simulink model "TestSeqAndDMS_Master"  (R2015b)
settings: Solver=FixedStepDiscrete  SolverMode=SingleTasking  StartTime=0.0  StopTime=inf  RelTol=1e-3
PreLoadFcn:
  | addpath RealTime_Pacer
PostLoadFcn:
  | StimuliImport
libraries: Word2Bytes_lib x41, simulink x3, instrumentlib x3, epoch_time_lib x2, realtime_pacer_lib x1
settings Model: Creator=ch24070  LastModifiedBy=ED12083
settings DataIOCC: LimitDataPoints=off  SaveFormat=StructureWithTime
settings DebuggingCC: SFUnexpectedBacktrackingDiag=error  SFNoUnconditionalDefaultTransitionDiag=error
settings HardwareCC: ProdWordSize=32  ProdHWDeviceType=Specified
settings ModelReferenceCC: PropagateSignalLabelsOutOfModel=on
settings GRTTargetCC: TargetLangStandard=C99 (ISO)
settings ConfigComp: CovMetricSettings=dwe  CovHtmlReporting=off  CovSaveCumulativeToWorkspaceVar=off  CovSaveSingleToWorkspaceVar=off  CovModelRefEnable=Off  CovExternalEMLEnable=on

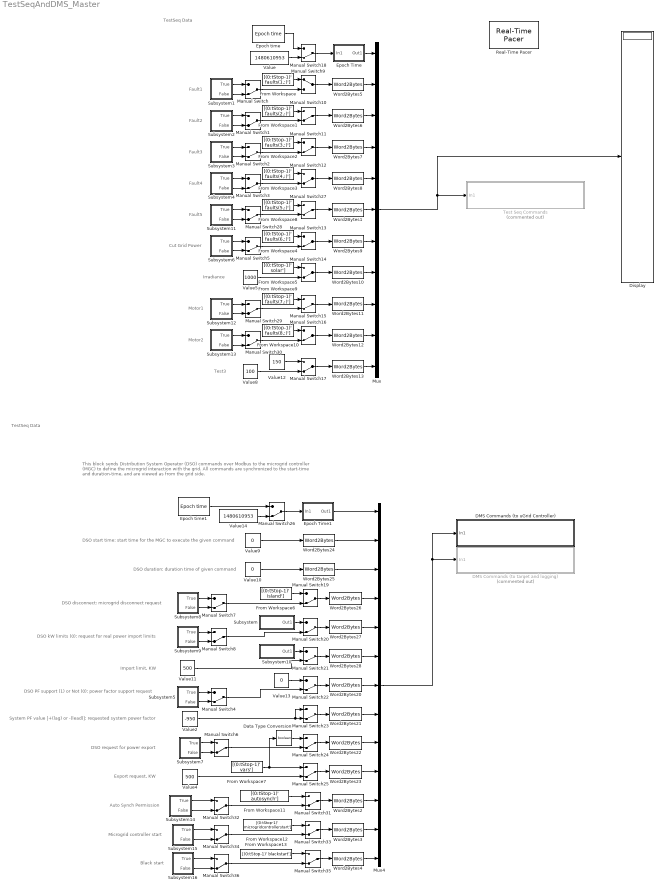
== system TestSeqAndDMS_Master ==
  note: Fault1
  note: This block sends Distribution System Operator (DSO) commands over Modbus to the microgrid controller (MGC) to define the microgrid
      | interaction with the grid. All commands are synchronized to the start-time and duration-time, and are viewed as from the grid side.
  note: TestSeq Data
  note: Fault2
  note: Fault3
  note: Fault4
  note: Cut Grid Power
  note: Irradiance
  note: Motor1
  note: Motor2
  note: Test3
  note: DSO disconnect: microgrid disconnect request
  note: DSO kW limits (0): request for real power import limits
  note: Import limit, KW
  note: DSO PF support (1) or Not (0): power factor support request
  note: System PF value [+(lag) or -(lead)]: requested system power factor
  note: DSO request for power export
  note: Export request, KW
  note: DSO start time: start time for the MGC to execute the given command
  note: DSO duration: duration time of given command
  note: Fault5
  note: Auto Synch Permission
  note: Microgrid controller start
  note: Black start
  note: TestSeq Data
  DMS Commands (to target and logging) : Subsystem  Commented=on  mask{destIP='192.168.10.54', unitID=54, modAddr=2000}
      mask prompts: destIP "Destination IP"; modAddr "Modbus Starting Address"
      mask Display:
      | text(5, 40, 'Modbus Master Write Holding Registers');
      | text(5, 20, ['Dest IP: ' destIP]);
  DMS Commands (to uGrid Controller) : Subsystem  mask{destIP='10.10.45.19', unitID=1, modAddr=2000}
      mask prompts: destIP "Destination IP"; modAddr "Modbus Starting Address"
      mask Display:
      | text(5, 40, 'Modbus Master Write Holding Registers');
      | text(5, 20, ['Dest IP: ' destIP]);
  Data Type Conversion : DataTypeConversion  OutDataTypeStr=boolean
  Display : Display
  Epoch Time : Subsystem
  Epoch Time1 : Subsystem
  Epoch time : epoch_time_lib/Epoch time  syncRate=10  clkRate=1
  Epoch time1 : epoch_time_lib/Epoch time  syncRate=10  clkRate=1
  From Workspace : FromWorkspace  VariableName=[(0:tStop-1)' faults(1,:)']  SampleTime=1  OutputAfterFinalValue=Holding final value
  From Workspace1 : FromWorkspace  VariableName=[(0:tStop-1)' faults(2,:)']  SampleTime=1  OutputAfterFinalValue=Holding final value
  From Workspace10 : FromWorkspace  VariableName=[(0:tStop-1)' faults(8,:)']  SampleTime=1  OutputAfterFinalValue=Holding final value
  From Workspace11 : FromWorkspace  VariableName=[(0:tStop-1)' autosynch']  SampleTime=1  OutputAfterFinalValue=Holding final value
  From Workspace12 : FromWorkspace  VariableName=[(0:tStop-1)' microgridcontrollerstart']  SampleTime=1  OutputAfterFinalValue=Holding final value
  From Workspace13 : FromWorkspace  VariableName=[(0:tStop-1)' blackstart']  SampleTime=1  OutputAfterFinalValue=Holding final value
  From Workspace2 : FromWorkspace  VariableName=[(0:tStop-1)' faults(3,:)']  SampleTime=1  OutputAfterFinalValue=Holding final value
  From Workspace3 : FromWorkspace  VariableName=[(0:tStop-1)' faults(4,:)']  SampleTime=1  OutputAfterFinalValue=Holding final value
  From Workspace4 : FromWorkspace  VariableName=[(0:tStop-1)' faults(6,:)']  SampleTime=1  OutputAfterFinalValue=Holding final value
  From Workspace5 : FromWorkspace  VariableName=[(0:tStop-1)' solar']  SampleTime=1  OutputAfterFinalValue=Holding final value
  From Workspace6 : FromWorkspace  VariableName=[(0:tStop-1)' island']  SampleTime=1  OutputAfterFinalValue=Holding final value
  From Workspace7 : FromWorkspace  VariableName=[(0:tStop-1)' vars']  SampleTime=1  OutputAfterFinalValue=Holding final value
  From Workspace8 : FromWorkspace  VariableName=[(0:tStop-1)' faults(5,:)']  SampleTime=1  OutputAfterFinalValue=Holding final value
  From Workspace9 : FromWorkspace  VariableName=[(0:tStop-1)' faults(7,:)']  SampleTime=1  OutputAfterFinalValue=Holding final value
  Manual Switch{,1..8,10..36} (36 alike) : ManualSwitch  CurrentSetting=0
  Manual Switch9 : ManualSwitch
  Mux : Mux  Inputs=11
  Mux4 : Mux  Inputs=13
  Real-Time Pacer : realtime_pacer_lib/Real-Time Pacer  simTimePerRealTime=1
  Subsystem : Subsystem
  Subsystem1 : Subsystem
  Subsystem10 : Subsystem
  Subsystem11 : Subsystem
  Subsystem12 : Subsystem
  Subsystem13 : Subsystem
  Subsystem14 : Subsystem
  Subsystem15 : Subsystem
  Subsystem16 : Subsystem
  Subsystem2 : Subsystem
  Subsystem3 : Subsystem
  Subsystem4 : Subsystem
  Subsystem5 : Subsystem
  Subsystem6 : Subsystem
  Subsystem7 : Subsystem
  Subsystem8 : Subsystem
  Subsystem9 : Subsystem
  Test Seq Commands : Subsystem  Commented=on  mask{destIP='192.168.10.56', unitID=56, modAddr=2000}
      mask prompts: destIP "Destination IP"; modAddr "Modbus Starting Address"
      mask Display:
      | text(5, 40, 'Modbus Master Write Holding Registers');
      | text(5, 20, ['Dest IP: ' destIP]);
  Value : Constant  Value=1480610953  OutDataTypeStr=uint32
  Value10 : Constant  Value=0  OutDataTypeStr=uint16
  Value11 : Constant  Value=500  OutDataTypeStr=uint16
  Value12 : Constant  Value=150  OutDataTypeStr=uint16
  Value13 : Constant  Value=0  OutDataTypeStr=uint16
  Value14 : Constant  Value=1480610953  OutDataTypeStr=uint32
  Value2 : Constant  Value=-950  OutDataTypeStr=int16
  Value4 : Constant  Value=500  OutDataTypeStr=uint16
  Value5 : Constant  Value=1000  OutDataTypeStr=uint16
  Value8 : Constant  Value=100  OutDataTypeStr=uint16
  Value9 : Constant  Value=0  OutDataTypeStr=uint16
  Word2Bytes{1..13,20..28} (22 alike) : Word2Bytes_lib/Word2Bytes
  wires:
  Epoch Time/1(Out1) -> Mux/1
  Subsystem1/2(False) -> Manual Switch/2
  Word2Bytes5/1 -> Mux/2
  Word2Bytes6/1 -> Mux/3
  Word2Bytes7/1 -> Mux/4
  Word2Bytes8/1 -> Mux/5
  Subsystem1/1(True) -> Manual Switch/1
  Subsystem2/2(False) -> Manual Switch1/2
  Subsystem2/1(True) -> Manual Switch1/1
  Subsystem3/2(False) -> Manual Switch2/2
  Subsystem3/1(True) -> Manual Switch2/1
  Subsystem4/1(True) -> Manual Switch3/1
  Subsystem6/2(False) -> Manual Switch5/2
  Subsystem6/1(True) -> Manual Switch5/1
  Subsystem4/2(False) -> Manual Switch3/2
  Epoch Time1/1(Out1) -> Mux4/1
  Value9/1 -> Word2Bytes24/1
  Word2Bytes24/1 -> Mux4/2
  Value10/1 -> Word2Bytes25/1
  Word2Bytes25/1 -> Mux4/3
  Word2Bytes26/1 -> Mux4/4
  Word2Bytes27/1 -> Mux4/5
  Word2Bytes28/1 -> Mux4/6
  Word2Bytes20/1 -> Mux4/7
  Word2Bytes21/1 -> Mux4/8
  Word2Bytes22/1 -> Mux4/9
  Word2Bytes23/1 -> Mux4/10
  Subsystem8/2(False) -> Manual Switch7/2
  Subsystem8/1(True) -> Manual Switch7/1
  Subsystem9/1(True) -> Manual Switch8/1
  Subsystem9/2(False) -> Manual Switch8/2
  Subsystem5/2(False) -> Manual Switch4/2
  Subsystem5/1(True) -> Manual Switch4/1
  Subsystem7/2(False) -> Manual Switch6/2
  Subsystem7/1(True) -> Manual Switch6/1
  Manual Switch9/1 -> Word2Bytes5/1
  Manual Switch/1 -> Manual Switch9/2
  Manual Switch10/1 -> Word2Bytes6/1
  Manual Switch11/1 -> Word2Bytes7/1
  Manual Switch12/1 -> Word2Bytes8/1
  Manual Switch13/1 -> Word2Bytes9/1
  Manual Switch14/1 -> Word2Bytes10/1
  Manual Switch15/1 -> Word2Bytes11/1
  Manual Switch16/1 -> Word2Bytes12/1
  Manual Switch17/1 -> Word2Bytes13/1
  Manual Switch1/1 -> Manual Switch10/2
  Manual Switch2/1 -> Manual Switch11/2
  Manual Switch3/1 -> Manual Switch12/2
  Manual Switch5/1 -> Manual Switch13/2
  Value5/1 -> Manual Switch14/2
  Manual Switch29/1 -> Manual Switch15/2
  Value8/1 -> Manual Switch17/2
  From Workspace/1 -> Manual Switch9/1
  From Workspace1/1 -> Manual Switch10/1
  From Workspace2/1 -> Manual Switch11/1
  From Workspace3/1 -> Manual Switch12/1
  From Workspace4/1 -> Manual Switch13/1
  From Workspace5/1 -> Manual Switch14/1
  Value12/1 -> Manual Switch17/1
  Manual Switch18/1 -> Epoch Time/1(In1)
  Value/1 -> Manual Switch18/2
  Epoch time/1 -> Manual Switch18/1
  Manual Switch19/1 -> Word2Bytes26/1
  From Workspace6/1 -> Manual Switch19/1
  Manual Switch7/1 -> Manual Switch19/2
  Manual Switch20/1 -> Word2Bytes27/1
  Manual Switch8/1 -> Manual Switch20/2
  Subsystem/1(Out1) -> Manual Switch20/1
  Subsystem10/1(Out1) -> Manual Switch21/1
  Manual Switch21/1 -> Word2Bytes28/1
  Value11/1 -> Manual Switch21/2
  Manual Switch22/1 -> Word2Bytes20/1
  Manual Switch4/1 -> Manual Switch22/2
  Value13/1 -> Manual Switch22/1
  Manual Switch23/1 -> Word2Bytes21/1
  Value2/1 -> Manual Switch23/1, Manual Switch23/2
  Manual Switch24/1 -> Word2Bytes22/1
  Manual Switch25/1 -> Word2Bytes23/1
  Value4/1 -> Manual Switch25/2
  From Workspace7/1 -> Data Type Conversion/1, Manual Switch25/1
  Manual Switch6/1 -> Manual Switch24/2
  Data Type Conversion/1 -> Manual Switch24/1
  Manual Switch26/1 -> Epoch Time1/1(In1)
  Value14/1 -> Manual Switch26/2
  Epoch time1/1 -> Manual Switch26/1
  Subsystem11/1(True) -> Manual Switch28/1
  Subsystem11/2(False) -> Manual Switch28/2
  Manual Switch27/1 -> Word2Bytes1/1
  Manual Switch28/1 -> Manual Switch27/2
  Word2Bytes1/1 -> Mux/6
  From Workspace8/1 -> Manual Switch27/1
  Word2Bytes9/1 -> Mux/7
  Word2Bytes10/1 -> Mux/8
  Word2Bytes11/1 -> Mux/9
  Word2Bytes12/1 -> Mux/10
  Word2Bytes13/1 -> Mux/11
  Mux/1 -> Display/1, Test Seq Commands/1(In1)
  Mux4/1 -> DMS Commands (to uGrid Controller)/1(In1), DMS Commands (to target and logging)/1(In1)
  Subsystem12/2(False) -> Manual Switch29/2
  Subsystem12/1(True) -> Manual Switch29/1
  Subsystem13/2(False) -> Manual Switch30/2
  Subsystem13/1(True) -> Manual Switch30/1
  Manual Switch30/1 -> Manual Switch16/2
  From Workspace9/1 -> Manual Switch15/1
  From Workspace10/1 -> Manual Switch16/1
  Manual Switch32/1 -> Manual Switch31/2
  Word2Bytes2/1 -> Mux4/11
  Subsystem14/1(True) -> Manual Switch32/1
  Subsystem14/2(False) -> Manual Switch32/2
  From Workspace11/1 -> Manual Switch31/1
  Manual Switch31/1 -> Word2Bytes2/1
  Manual Switch34/1 -> Manual Switch33/2
  Word2Bytes3/1 -> Mux4/12
  Subsystem15/1(True) -> Manual Switch34/1
  Subsystem15/2(False) -> Manual Switch34/2
  From Workspace12/1 -> Manual Switch33/1
  Manual Switch33/1 -> Word2Bytes3/1
  Manual Switch36/1 -> Manual Switch35/2
  Word2Bytes4/1 -> Mux4/13
  Subsystem16/1(True) -> Manual Switch36/1
  Subsystem16/2(False) -> Manual Switch36/2
  Manual Switch35/1 -> Word2Bytes4/1
  From Workspace13/1 -> Manual Switch35/1

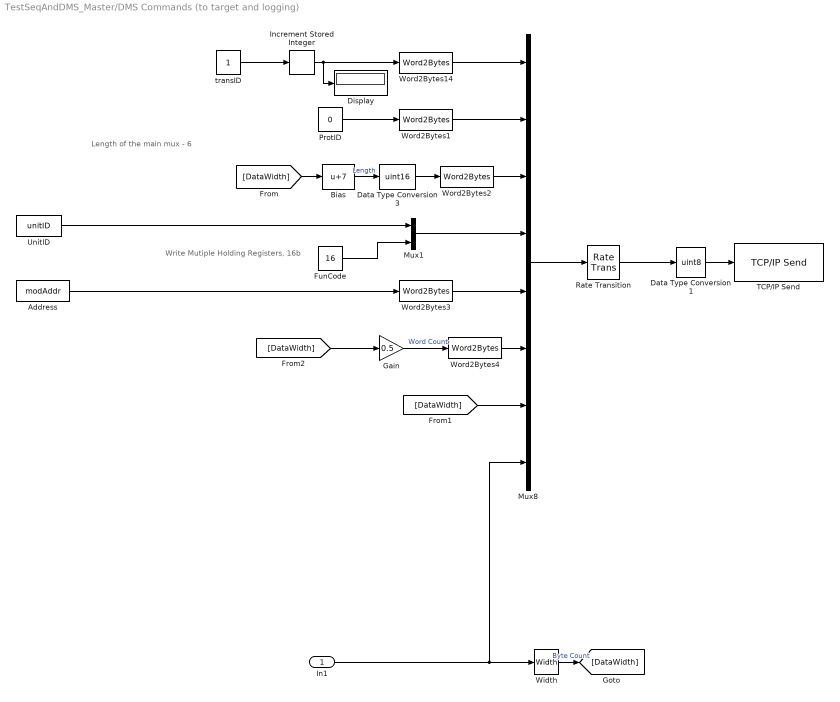
== system TestSeqAndDMS_Master/DMS Commands (to target and logging) ==
  note: Length of the main mux - 6
  note: Write Mutiple Holding Registers, 16b
  In1 : Inport
  Address : Constant  Value=modAddr  OutDataTypeStr=uint16
  Bias : Bias  Bias=7
  Data Type Conversion1 : DataTypeConversion  OutDataTypeStr=uint8  ConvertRealWorld=Stored Integer (SI)  RndMeth=Nearest
  Data Type Conversion3 : DataTypeConversion  OutDataTypeStr=uint16
  Display : Display
  FunCode : Constant  Value=16  OutDataTypeStr=uint8
  Gain : Gain  Gain=0.5  OutDataTypeStr=uint16  RndMeth=Ceiling
  Increment Stored Integer : simulink/Additional Math & Discrete/Additional Math: Increment - Decrement/Increment Stored Integer
  Mux1 : Mux  Inputs=2
  Mux8 : Mux  Inputs=8
  ProtID : Constant  Value=0  OutDataTypeStr=uint16
  Rate Transition : RateTransition  OutPortSampleTime=0.5
  TCP/IP Send : instrumentlib/TCP//IP Send  Priority=1  Host=192.168.10.54  Port=502  EnableBlockingMode=off  Timeout=10  ByteOrder=BigEndian
  UnitID : Constant  Value=unitID  OutDataTypeStr=uint8
  Width : Width  DataType=uint8
  Word2Bytes{1..4,14} (5 alike) : Word2Bytes_lib/Word2Bytes
  transID : Constant  OutDataTypeStr=uint16
  wires:
  Mux8/1 -> Rate Transition/1
  Data Type Conversion1/1 -> TCP/IP Send/1
  Address/1 -> Word2Bytes3/1
  Bias/1 -> Data Type Conversion3/1  "Length"
  ProtID/1 -> Word2Bytes1/1
  Rate Transition/1 -> Data Type Conversion1/1
  Increment Stored Integer/1 -> Display/1, Word2Bytes14/1
  Mux1/1 -> Mux8/4
  UnitID/1 -> Mux1/1
  FunCode/1 -> Mux1/2
  transID/1 -> Increment Stored Integer/1
  Word2Bytes14/1 -> Mux8/1
  Word2Bytes1/1 -> Mux8/2
  Word2Bytes2/1 -> Mux8/3
  Word2Bytes3/1 -> Mux8/5
  Gain/1 -> Word2Bytes4/1  "Word Count"
  Word2Bytes4/1 -> Mux8/6
  In1/1 -> Width/1, Mux8/8
  Width/1 -> [DataWidth]  "Byte Count"
  [DataWidth] -> Mux8/7
  [DataWidth] -> Gain/1
  [DataWidth] -> Bias/1
  Data Type Conversion3/1 -> Word2Bytes2/1

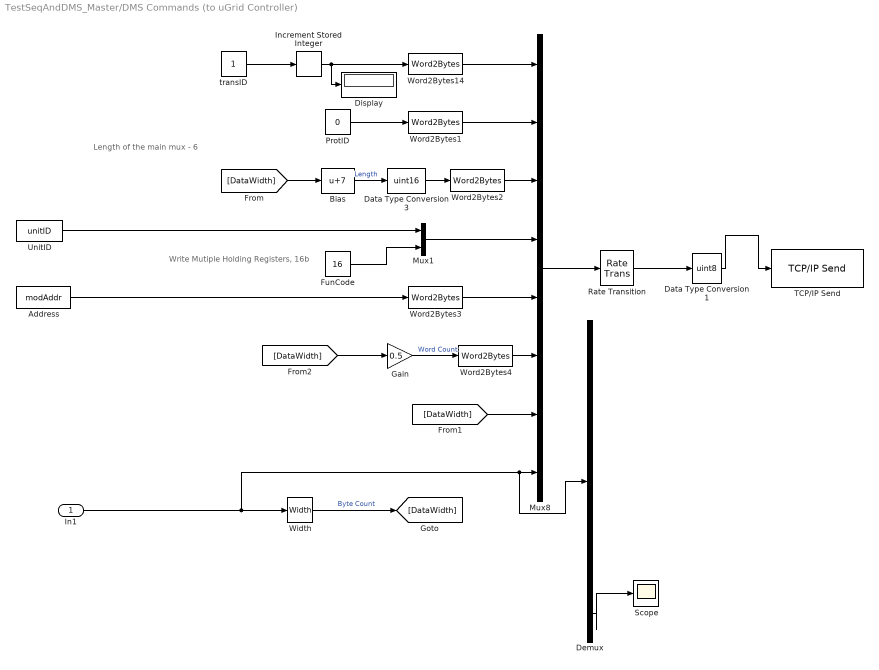
== system TestSeqAndDMS_Master/DMS Commands (to uGrid Controller) ==
  note: Write Mutiple Holding Registers, 16b
  note: Length of the main mux - 6
  In1 : Inport
  Address : Constant  Value=modAddr  OutDataTypeStr=uint16
  Bias : Bias  Bias=7
  Data Type Conversion1 : DataTypeConversion  OutDataTypeStr=uint8  ConvertRealWorld=Stored Integer (SI)  RndMeth=Nearest
  Data Type Conversion3 : DataTypeConversion  OutDataTypeStr=uint16
  Demux : Demux  Outputs=28
  Display : Display
  FunCode : Constant  Value=16  OutDataTypeStr=uint8
  Gain : Gain  Gain=0.5  OutDataTypeStr=uint16  RndMeth=Ceiling
  Increment Stored Integer : simulink/Additional Math & Discrete/Additional Math: Increment - Decrement/Increment Stored Integer
  Mux1 : Mux  Inputs=2
  Mux8 : Mux  Inputs=8
  ProtID : Constant  Value=0  OutDataTypeStr=uint16
  Rate Transition : RateTransition  OutPortSampleTime=0.1
  Scope : Scope
  TCP/IP Send : instrumentlib/TCP//IP Send  Priority=1  Host=10.10.45.19  Port=502  EnableBlockingMode=off  Timeout=10  ByteOrder=BigEndian
  UnitID : Constant  Value=unitID  OutDataTypeStr=uint8
  Width : Width  DataType=uint8
  Word2Bytes{1..4,14} (5 alike) : Word2Bytes_lib/Word2Bytes
  transID : Constant  OutDataTypeStr=uint16
  wires:
  Data Type Conversion3/1 -> Word2Bytes2/1
  [DataWidth] -> Bias/1
  [DataWidth] -> Gain/1
  [DataWidth] -> Mux8/7
  Width/1 -> [DataWidth]  "Byte Count"
  In1/1 -> Demux/1, Mux8/8, Width/1
  Word2Bytes4/1 -> Mux8/6
  Gain/1 -> Word2Bytes4/1  "Word Count"
  Word2Bytes3/1 -> Mux8/5
  Word2Bytes2/1 -> Mux8/3
  Word2Bytes1/1 -> Mux8/2
  Word2Bytes14/1 -> Mux8/1
  transID/1 -> Increment Stored Integer/1
  FunCode/1 -> Mux1/2
  UnitID/1 -> Mux1/1
  Mux1/1 -> Mux8/4
  Increment Stored Integer/1 -> Word2Bytes14/1, Display/1
  Rate Transition/1 -> Data Type Conversion1/1
  ProtID/1 -> Word2Bytes1/1
  Bias/1 -> Data Type Conversion3/1  "Length"
  Address/1 -> Word2Bytes3/1
  Data Type Conversion1/1 -> TCP/IP Send/1
  Mux8/1 -> Rate Transition/1
  Demux/26 -> Scope/1

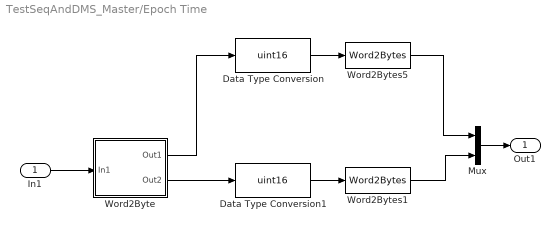
== system TestSeqAndDMS_Master/Epoch Time ==
  In1 : Inport
  Data Type Conversion : DataTypeConversion  OutDataTypeStr=uint16
  Data Type Conversion1 : DataTypeConversion  OutDataTypeStr=uint16
  Mux : Mux  Inputs=2
  Word2Byte : Subsystem
  Word2Bytes1 : Word2Bytes_lib/Word2Bytes
  Word2Bytes5 : Word2Bytes_lib/Word2Bytes
  Out1 : Outport
  wires:
  Data Type Conversion1/1 -> Word2Bytes1/1
  Word2Byte/2(Out2) -> Data Type Conversion1/1
  In1/1 -> Word2Byte/1(In1)
  Word2Byte/1(Out1) -> Data Type Conversion/1
  Data Type Conversion/1 -> Word2Bytes5/1
  Mux/1 -> Out1/1
  Word2Bytes5/1 -> Mux/1
  Word2Bytes1/1 -> Mux/2

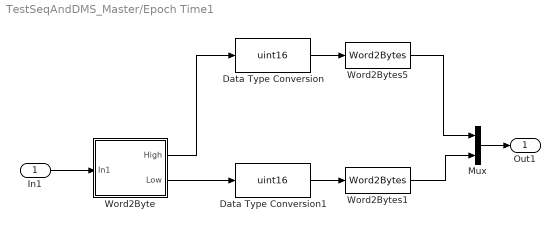
== system TestSeqAndDMS_Master/Epoch Time1 ==
  In1 : Inport
  Data Type Conversion : DataTypeConversion  OutDataTypeStr=uint16
  Data Type Conversion1 : DataTypeConversion  OutDataTypeStr=uint16
  Mux : Mux  Inputs=2
  Word2Byte : Subsystem
  Word2Bytes1 : Word2Bytes_lib/Word2Bytes
  Word2Bytes5 : Word2Bytes_lib/Word2Bytes
  Out1 : Outport
  wires:
  Data Type Conversion1/1 -> Word2Bytes1/1
  Word2Byte/2(Low) -> Data Type Conversion1/1
  In1/1 -> Word2Byte/1(In1)
  Word2Byte/1(High) -> Data Type Conversion/1
  Data Type Conversion/1 -> Word2Bytes5/1
  Mux/1 -> Out1/1
  Word2Bytes5/1 -> Mux/1
  Word2Bytes1/1 -> Mux/2

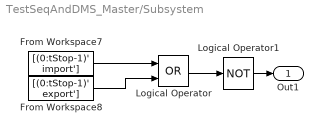
== system TestSeqAndDMS_Master/Subsystem ==
  From Workspace7 : FromWorkspace  VariableName=[(0:tStop-1)' import']  SampleTime=1  OutputAfterFinalValue=Holding final value
  From Workspace8 : FromWorkspace  VariableName=[(0:tStop-1)' export']  SampleTime=1  OutputAfterFinalValue=Holding final value
  Logical Operator : Logic  Operator=OR  AllPortsSameDT=off  OutDataTypeStr=boolean
  Logical Operator1 : Logic  Operator=NOT  AllPortsSameDT=off  OutDataTypeStr=boolean
  Out1 : Outport
  wires:
  Logical Operator1/1 -> Out1/1
  Logical Operator/1 -> Logical Operator1/1
  From Workspace8/1 -> Logical Operator/2
  From Workspace7/1 -> Logical Operator/1

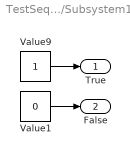
== system TestSeqAndDMS_Master/Subsystem1 ==
  Value1 : Constant  Value=0  OutDataTypeStr=uint16
  Value9 : Constant  OutDataTypeStr=uint16
  True : Outport
  False : Outport  Port=2
  wires:
  Value9/1 -> True/1
  Value1/1 -> False/1

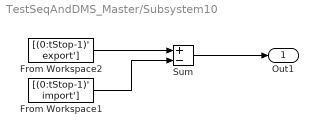
== system TestSeqAndDMS_Master/Subsystem10 ==
  From Workspace1 : FromWorkspace  VariableName=[(0:tStop-1)' import']  SampleTime=1  OutputAfterFinalValue=Holding final value
  From Workspace2 : FromWorkspace  VariableName=[(0:tStop-1)' export']  SampleTime=1  OutputAfterFinalValue=Holding final value
  Sum : Sum  Inputs=+-
  Out1 : Outport
  wires:
  Sum/1 -> Out1/1
  From Workspace2/1 -> Sum/1
  From Workspace1/1 -> Sum/2

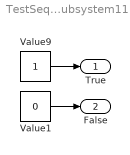
== system TestSeqAndDMS_Master/Subsystem11 ==
  Value1 : Constant  Value=0  OutDataTypeStr=uint16
  Value9 : Constant  OutDataTypeStr=uint16
  True : Outport
  False : Outport  Port=2
  wires:
  Value9/1 -> True/1
  Value1/1 -> False/1

== system TestSeqAndDMS_Master/Subsystem12 ==
  Value1 : Constant  Value=0  OutDataTypeStr=uint16
  Value9 : Constant  OutDataTypeStr=uint16
  True : Outport
  False : Outport  Port=2
  wires:
  Value9/1 -> True/1
  Value1/1 -> False/1

== system TestSeqAndDMS_Master/Subsystem13 ==
  Value1 : Constant  Value=0  OutDataTypeStr=uint16
  Value9 : Constant  OutDataTypeStr=uint16
  True : Outport
  False : Outport  Port=2
  wires:
  Value1/1 -> False/1
  Value9/1 -> True/1

== system TestSeqAndDMS_Master/Subsystem14 ==
  Value1 : Constant  Value=0  OutDataTypeStr=uint16
  Value9 : Constant  OutDataTypeStr=uint16
  True : Outport
  False : Outport  Port=2
  wires:
  Value9/1 -> True/1
  Value1/1 -> False/1

== system TestSeqAndDMS_Master/Subsystem15 ==
  Value1 : Constant  Value=0  OutDataTypeStr=uint16
  Value9 : Constant  OutDataTypeStr=uint16
  True : Outport
  False : Outport  Port=2
  wires:
  Value9/1 -> True/1
  Value1/1 -> False/1

== system TestSeqAndDMS_Master/Subsystem16 ==
  Value1 : Constant  Value=0  OutDataTypeStr=uint16
  Value9 : Constant  OutDataTypeStr=uint16
  True : Outport
  False : Outport  Port=2
  wires:
  Value9/1 -> True/1
  Value1/1 -> False/1

== system TestSeqAndDMS_Master/Subsystem2 ==
  Value1 : Constant  Value=0  OutDataTypeStr=uint16
  Value9 : Constant  OutDataTypeStr=uint16
  True : Outport
  False : Outport  Port=2
  wires:
  Value9/1 -> True/1
  Value1/1 -> False/1

== system TestSeqAndDMS_Master/Subsystem3 ==
  Value1 : Constant  Value=0  OutDataTypeStr=uint16
  Value9 : Constant  OutDataTypeStr=uint16
  True : Outport
  False : Outport  Port=2
  wires:
  Value9/1 -> True/1
  Value1/1 -> False/1

== system TestSeqAndDMS_Master/Subsystem4 ==
  Value1 : Constant  Value=0  OutDataTypeStr=uint16
  Value9 : Constant  OutDataTypeStr=uint16
  True : Outport
  False : Outport  Port=2
  wires:
  Value9/1 -> True/1
  Value1/1 -> False/1

== system TestSeqAndDMS_Master/Subsystem5 ==
  Value1 : Constant  Value=0  OutDataTypeStr=uint16
  Value9 : Constant  OutDataTypeStr=uint16
  True : Outport
  False : Outport  Port=2
  wires:
  Value1/1 -> False/1
  Value9/1 -> True/1

== system TestSeqAndDMS_Master/Subsystem6 ==
  Value1 : Constant  Value=0  OutDataTypeStr=uint16
  Value9 : Constant  OutDataTypeStr=uint16
  True : Outport
  False : Outport  Port=2
  wires:
  Value1/1 -> False/1
  Value9/1 -> True/1

== system TestSeqAndDMS_Master/Subsystem7 ==
  Value1 : Constant  Value=0  OutDataTypeStr=uint16
  Value9 : Constant  OutDataTypeStr=uint16
  True : Outport
  False : Outport  Port=2
  wires:
  Value9/1 -> True/1
  Value1/1 -> False/1

== system TestSeqAndDMS_Master/Subsystem8 ==
  Value1 : Constant  Value=0  OutDataTypeStr=uint16
  Value9 : Constant  OutDataTypeStr=uint16
  True : Outport
  False : Outport  Port=2
  wires:
  Value9/1 -> True/1
  Value1/1 -> False/1

== system TestSeqAndDMS_Master/Subsystem9 ==
  Value1 : Constant  Value=0  OutDataTypeStr=uint16
  Value9 : Constant  OutDataTypeStr=uint16
  True : Outport
  False : Outport  Port=2
  wires:
  Value9/1 -> True/1
  Value1/1 -> False/1

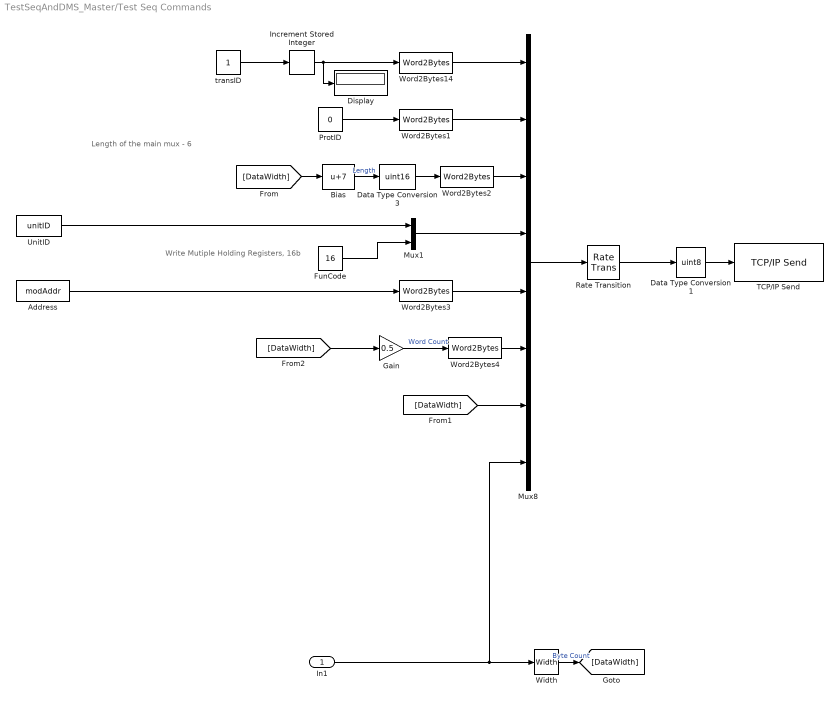
== system TestSeqAndDMS_Master/Test Seq Commands ==
  note: Length of the main mux - 6
  note: Write Mutiple Holding Registers, 16b
  In1 : Inport
  Address : Constant  Value=modAddr  OutDataTypeStr=uint16
  Bias : Bias  Bias=7
  Data Type Conversion1 : DataTypeConversion  OutDataTypeStr=uint8  ConvertRealWorld=Stored Integer (SI)  RndMeth=Nearest
  Data Type Conversion3 : DataTypeConversion  OutDataTypeStr=uint16
  Display : Display
  FunCode : Constant  Value=16  OutDataTypeStr=uint8
  Gain : Gain  Gain=0.5  OutDataTypeStr=uint16  RndMeth=Ceiling
  Increment Stored Integer : simulink/Additional Math & Discrete/Additional Math: Increment - Decrement/Increment Stored Integer
  Mux1 : Mux  Inputs=2
  Mux8 : Mux  Inputs=8
  ProtID : Constant  Value=0  OutDataTypeStr=uint16
  Rate Transition : RateTransition  OutPortSampleTime=0.5
  TCP/IP Send : instrumentlib/TCP//IP Send  Priority=1  Host=192.168.10.56  Port=502  EnableBlockingMode=off  Timeout=10  ByteOrder=BigEndian
  UnitID : Constant  Value=unitID  OutDataTypeStr=uint8
  Width : Width  DataType=uint8
  Word2Bytes{1..4,14} (5 alike) : Word2Bytes_lib/Word2Bytes
  transID : Constant  OutDataTypeStr=uint16
  wires:
  Mux8/1 -> Rate Transition/1
  Data Type Conversion1/1 -> TCP/IP Send/1
  Address/1 -> Word2Bytes3/1
  Bias/1 -> Data Type Conversion3/1  "Length"
  ProtID/1 -> Word2Bytes1/1
  Rate Transition/1 -> Data Type Conversion1/1
  Increment Stored Integer/1 -> Display/1, Word2Bytes14/1
  Mux1/1 -> Mux8/4
  UnitID/1 -> Mux1/1
  FunCode/1 -> Mux1/2
  transID/1 -> Increment Stored Integer/1
  Word2Bytes14/1 -> Mux8/1
  Word2Bytes1/1 -> Mux8/2
  Word2Bytes2/1 -> Mux8/3
  Word2Bytes3/1 -> Mux8/5
  Gain/1 -> Word2Bytes4/1  "Word Count"
  Word2Bytes4/1 -> Mux8/6
  In1/1 -> Width/1, Mux8/8
  Width/1 -> [DataWidth]  "Byte Count"
  [DataWidth] -> Mux8/7
  [DataWidth] -> Gain/1
  [DataWidth] -> Bias/1
  Data Type Conversion3/1 -> Word2Bytes2/1

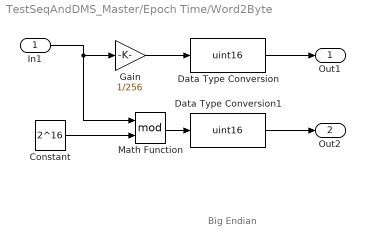
== system TestSeqAndDMS_Master/Epoch Time/Word2Byte ==
  note: Big Endian
  In1 : Inport
  Constant : Constant  Value=2^16  OutDataTypeStr=Inherit: Inherit via back propagation
  Data Type Conversion : DataTypeConversion  OutDataTypeStr=uint16
  Data Type Conversion1 : DataTypeConversion  OutDataTypeStr=uint16
  Gain : Gain  Gain=1/256
  Math Function : Math  Operator=mod  SaturateOnIntegerOverflow=on
  Out1 : Outport
  Out2 : Outport  Port=2
  wires:
  Gain/1 -> Data Type Conversion/1
  Constant/1 -> Math Function/2
  In1/1 -> Math Function/1, Gain/1
  Math Function/1 -> Data Type Conversion1/1
  Data Type Conversion/1 -> Out1/1
  Data Type Conversion1/1 -> Out2/1

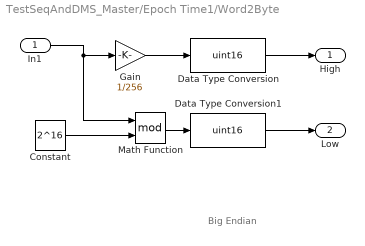
== system TestSeqAndDMS_Master/Epoch Time1/Word2Byte ==
  note: Big Endian
  In1 : Inport
  Constant : Constant  Value=2^16  OutDataTypeStr=Inherit: Inherit via back propagation
  Data Type Conversion : DataTypeConversion  OutDataTypeStr=uint16
  Data Type Conversion1 : DataTypeConversion  OutDataTypeStr=uint16
  Gain : Gain  Gain=1/256
  Math Function : Math  Operator=mod  SaturateOnIntegerOverflow=on
  High : Outport
  Low : Outport  Port=2
  wires:
  Gain/1 -> Data Type Conversion/1
  Constant/1 -> Math Function/2
  In1/1 -> Math Function/1, Gain/1
  Math Function/1 -> Data Type Conversion1/1
  Data Type Conversion/1 -> High/1
  Data Type Conversion1/1 -> Low/1
